simulink model "nuclear"  (Simulink 7.8)
settings: Solver=ode45  StartTime=0.0  StopTime=24  RelTol=1e-3
libraries: simulink x2
settings Model: Creator=John  LastModifiedBy=John
settings DebuggingCC: SolverPrmCheckMsg=none

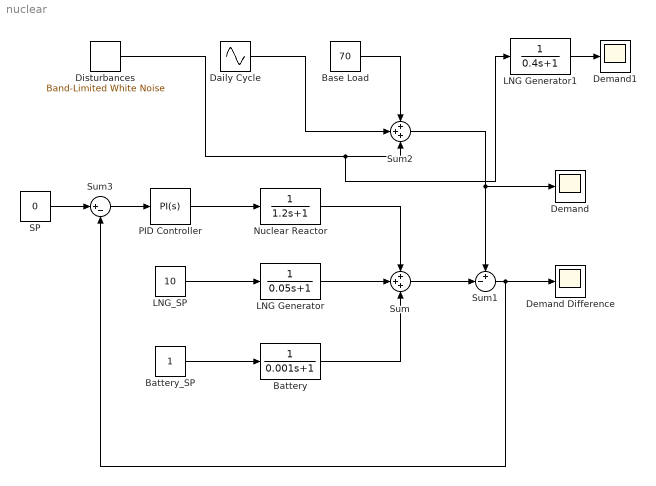
== system nuclear ==
  Base Load : Constant  Value=70
  Battery : TransferFcn  Denominator=[0.001 1]
  Battery_SP : Constant
  Daily Cycle : Sin  Amplitude=20  Frequency=2*3.1415/24  SampleTime=0
  Demand : Scope
  Demand Difference : Scope
  Demand1 : Scope
      settings: SaveName=ScopeData2
  Disturbances : simulink/Sources/Band-Limited White Noise  Cov=[5]  Ts=0.5  seed=[23342]
  LNG Generator : TransferFcn  Denominator=[0.05 1]
  LNG Generator1 : TransferFcn  Denominator=[0.4 1]
  LNG_SP : Constant  Value=10
  Nuclear Reactor : TransferFcn  Denominator=[1.2 1]
  PID Controller : simulink/Continuous/PID Controller  Controller=PI  TimeDomain=Continuous-time  SampleTime=1  IntegratorMethod=Forward Euler  FilterMethod=Forward Euler  Form=Parallel  P=-1  I=-1  D=0  N=100  InitialConditionSource=internal  InitialConditionForIntegrator=0  InitialConditionForFilter=0  ExternalReset=none  LimitOutput=on  UpperSaturationLimit=100  LowerSaturationLimit=0  LinearizeAsGain=off  AntiWindupMode=clamping  Kb=1  TrackingMode=off  Kt=1  PParamMin=[]  PParamMax=[]  IParamMin=[]  IParamMax=[]  DParamMin=[]  DParamMax=[]  NParamMin=[]  NParamMax=[]  KbParamMin=[]  KbParamMax=[]  KtParamMin=[]  KtParamMax=[]  POutMin=[]  POutMax=[]  IOutMin=[]  IOutMax=[]  DOutMin=[]  DOutMax=[]  NOutMin=[]  NOutMax=[]  KbOutMin=[]  KbOutMax=[]  KtOutMin=[]  KtOutMax=[]  IntegratorOutMin=[]  IntegratorOutMax=[]  FilterOutMin=[]  FilterOutMax=[]  SumOutMin=[]  SumOutMax=[]  SumI1OutMin=[]  SumI1OutMax=[]  SumI2OutMin=[]  SumI2OutMax=[]  SumI3OutMin=[]  SumI3OutMax=[]  SumDOutMin=[]  SumDOutMax=[]  SaturationOutMin=[]  SaturationOutMax=[]  IntegratorContinuousStateAttributes=''  IntegratorStateMustResolveToSignalObject=off  IntegratorRTWStateStorageClass=Auto  FilterContinuousStateAttributes=''  FilterStateMustResolveToSignalObject=off  FilterRTWStateStorageClass=Auto
  SP : Constant  Value=0
  Sum : Sum  Inputs=+++
  Sum1 : Sum  Inputs=+-|
  Sum2 : Sum  Inputs=+++
  Sum3 : Sum  Inputs=|+-
  wires:
  Nuclear Reactor/1 -> Sum/1
  LNG_SP/1 -> LNG Generator/1
  LNG Generator/1 -> Sum/2
  Battery_SP/1 -> Battery/1
  Battery/1 -> Sum/3
  Sum/1 -> Sum1/2
  Sum1/1 -> Demand Difference/1, Sum3/2
  Base Load/1 -> Sum2/1
  Daily Cycle/1 -> Sum2/2
  Sum2/1 -> Sum1/1, Demand/1
  PID Controller/1 -> Nuclear Reactor/1
  SP/1 -> Sum3/1
  Sum3/1 -> PID Controller/1
  Disturbances/1 -> Sum2/3, LNG Generator1/1
  LNG Generator1/1 -> Demand1/1
